simulink model "test_mux_parallel_charts"  (R2021b)
settings: Solver=VariableStepAuto  StartTime=0.0  StopTime=10.0  RelTol=1e-3
settings Model: Creator=grodriguez  LastModifiedBy=grodriguez

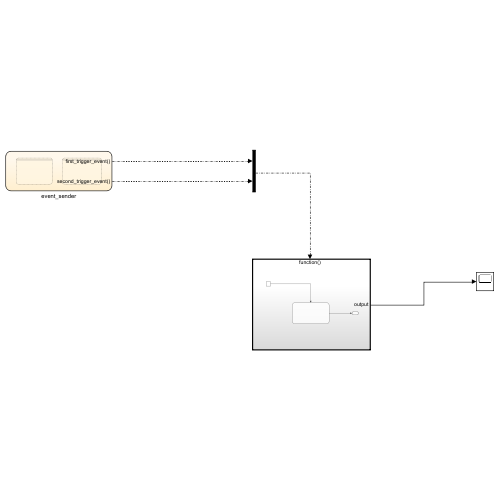
[thumbnail: Simulink's stored preview of the top-level diagram]
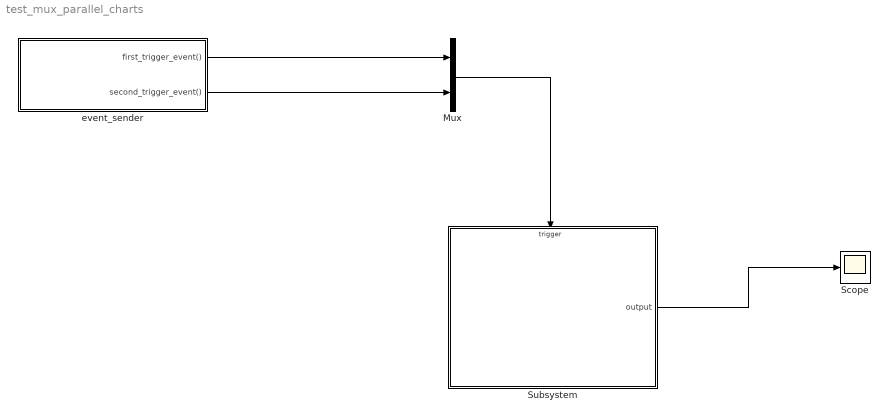
== system test_mux_parallel_charts ==
  Mux : Mux  Inputs=2
  Scope : Scope
  Subsystem : Subsystem
  event_sender : Stateflow chart  TreatAsAtomicUnit=on
  wires:
  Mux/1 -> Subsystem/Trigger
  Subsystem/1(output) -> Scope/1
  event_sender/1(first_trigger_event()) -> Mux/1
  event_sender/2(second_trigger_event()) -> Mux/2

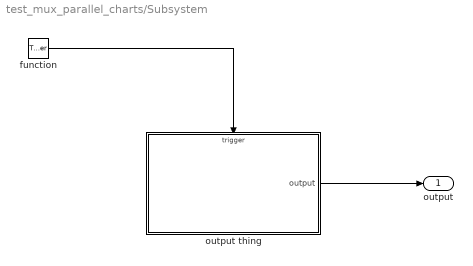
== system test_mux_parallel_charts/Subsystem ==
  function : TriggerPort  TriggerType=function-call  VariantControl=(inherit)  ShowOutputPort=on
  output thing : Stateflow chart  TreatAsAtomicUnit=on
  output : Outport
  wires:
  output thing/1(output) -> output/1
  function/1 -> output thing/Trigger

== stateflow chart test_mux_parallel_charts/Subsystem/output thing ==
  state state_3
    entry:
    output = -10;
  state state_1
    entry:
    output = output + 1;
  state state_2
    entry:
    output = output + 1;
  (default) -> state_1
  (junction 27) -> state_3
  state_1 -> (junction 27) [order 2] : second_trigger_event
  state_1 -> state_2 [order 1] : first_trigger_event
  (junction 11) -> state_1
  state_2 -> (junction 9) : second_trigger_event
  (junction 9) -> (junction 11)
  data: output output =0
  events: first_trigger_event input RISING_EDGE_EVENT; second_trigger_event input RISING_EDGE_EVENT

== stateflow chart test_mux_parallel_charts/event_sender ==
  state first_event [parallel]
    settings: executionOrder=1
    state init
    (default) -> (junction 14)
    (junction 14) -> (junction 18)
    (junction 21) -> (junction 18)
    (junction 16) -> (junction 21)
    (junction 18) -> first_event.init : {send(first_trigger_event);}
    first_event.init -> (junction 16)
  state second_event [parallel]
    settings: executionOrder=2
    state init
    (default) -> (junction 28)
    (junction 28) -> (junction 32)
    (junction 26) -> (junction 32)
    (junction 30) -> (junction 26)
    (junction 32) -> second_event.init : {send(second_trigger_event);}
    second_event.init -> (junction 30)
  events: first_trigger_event output FUNCTION_CALL_EVENT; second_trigger_event output FUNCTION_CALL_EVENT
